simulink model "VehicleDynamics3D"  (R2019b)
settings: Solver=ode15s  StartTime=0.0  StopTime=StopTime  FixedStep=.001  MaxStep=maxStep  RelTol=relTol  AbsTol=absTol  EnableMultiTasking=on
PreLoadFcn:
  | VehicleDynamicsInitialization
model workspace: external: MATLAB File sm_suspension_templates_params.m (data not in the file)
values from neighbouring files (symbols this model uses):
  followerCameraX = 7.5    [VehicleDynamicsInitialization.m]
  followerCameraZ = 3    [VehicleDynamicsInitialization.m]
  frontCameraX = -1.75    [VehicleDynamicsInitialization.m]
  frontCameraZ = 0.35    [VehicleDynamicsInitialization.m]
  isoCameraAimX = (1/2)*wheelbase    (= 0.75)    [VehicleDynamicsInitialization.m]
  isoCameraX = -3.1    [VehicleDynamicsInitialization.m]
  isoCameraY = 3.5    [VehicleDynamicsInitialization.m]
  isoCameraZ = 1.5    [VehicleDynamicsInitialization.m]
  Load = 200    [VehicleDynamicsInitialization.m]
  maxSteeringDisplacement = 10    [VehicleDynamicsInitialization.m]
  minSteeringDisplacement = -10    [VehicleDynamicsInitialization.m]
  SetPaceSampleTime = 0.1    [VehicleDynamicsInitialization.m]
  steeringInput = 0    [VehicleDynamicsInitialization.m]
  vehicleSpeed_kph = 0    [VehicleDynamicsInitialization.m]
  wheelbase = 1.5    [VehicleDynamicsInitialization.m]
undefined symbols (not defined in the file or in its folder): dwb, Floor, sigbuilder_block, wheel, X, Y, Z
libraries: sm_lib x195, sm_suspension_templates_lib x34, nesl_utility x15, Contact_Forces_Lib x4, simulink x2, fl_ps_legacy_lib x1, aerolibanimutils x1
(part 6 of 8)

== system VehicleDynamics3D/RearSuspension/L Suspension Assembly ==
  Knuckle : Subsystem  mask(Steering knuckle){H=dwb.knuckle.height, L=dwb.knuckle.length, T=dwb.knuckle.thickness, Wpr=dwb.knuckle.wheelattachprojwidth, Hpr=dwb.knuckle.wheelattachprojheight, Wc=dwb.knuckle.wishboneconnectorwidth, Rd=dwb.knuckle.driveshaftradius, Hd=dwb.knuckle.driveshaftheight, Rr=dwb.knuckle.chamferradius, Rt=dwb.knuckle.transitionradius, Rb=dwb.knuckle.ball.radius, Rp=dwb.knuckle.pin.radius, Hp=dwb.knuckle.pin.height, Ls=dwb.knuckle.steerarm.length, Ws=dwb.knuckle.steerarm.width, Ts=dwb.knuckle.steerarm.thickness, Hsf=dwb.knuckle.steerarm.forkheight, Lsf=dwb.knuckle.steerarm.forklength, Osf=dwb.knuckle.steerarm.forkoffset, Rsp=dwb.knuckle.pinradius, Rsr=dwb.knuckle.chamferradius, Rev=on, rho=dwb.knuckle.density, clr=dwb.knuckle.color}
      mask prompts: H "Height (cm):"; L "Length (cm):"; T "Thickness (cm):"; Wpr "Width of wheel attach projection (cm):"; Hpr "Height of wheel attach projection (cm):"; Wc "Width of wishbone connectors (cm):"; Rd "Drive shaft hole radius (cm):"; Hd "Drive shaft bearing housing height (cm):"; Rr "Chamfer/fillet radius (cm):"; Rt "Transition radius to wheel attach projection (cm):"; Rb "Ball radius (cm):"; Rp "Pin radius (cm):"; Hp "Pin height (cm):"; Ls "Length of arm (cm):"; Ws "Width of arm (cm):"; Ts "Thickness of arm (cm):"; Hsf "Height of forked section (cm):"; Lsf "Length of forked section (cm):"; Osf "Offset of forked section (cm):"; Rsp "Pin radius (cm):"; Rsr "Chamfer/fillet radius (cm):"; Rev "Reverse direction:"; rho "Density (kg/m^3):"; clr "Color ([r g b]):"
      mask help: This block models a steering knuckle. The wheel hub attaches to the steering knuckle. The steering knuckle attaches to the wishbone links. The ports U and D correspond to the frames where the knuckle connects to the wishbone links. The port W corresponds to the frame where the wheel hub attaches to the knuckle. The knuckle also has a rigidly attached steering arm that attaches to the steering rack via tie rods. The port S corresponds to the frame where the steering arm attaches to the tie rod.
      mask init:
      | s_knuckle_xsec = [0 -Hd/2; 0 -Hpr/2; Wpr -Hpr/2; Wpr -H/2;
      |                 Wpr+Wc -H/2; Wpr+Wc -H/2+T; Wpr+T -H/2+T;
      |                  Wpr+T -Hd/2];
      | 
      | s_knuckle_xsec = simmechanics.demohelpers.round_corners(s_knuckle_xsec, 2:7, ...
      |                              [Rr Rt Rr*ones(1,4)], 20);
      | 
      | n_knuckle_xsec = flipud([s_knuckle_xsec(:,1) -s_knuckle_xsec(:,2)]);                         
      | 
      | Roh = sqrt((L/2)^2 + (Hd/2)^2);
      | phi = atan2(Hd,L);
      | theta = linspace(pi/2-phi,pi/2+phi,50)';
      | sh_xsec = [Roh*cos(theta) Roh*sin(theta)];
      | theta = linspace(3*pi/2-phi,3*pi/2+phi,50)';
      | sh_xsec = [sh_xsec; Roh*cos(theta) Roh*sin(theta)];
      | theta = linspace(5*pi/2-phi,pi/2-phi,100)';
      | sh_xsec = [sh_xsec; sh_xsec(1,:); Rd*cos(theta) Rd*sin(theta)];
      | 
      | % Convert Rev variable into +/- 1 instead of 0 or 1
      | sgn = (2*Rev-1);
      mask DialogControl ParameterTabVar0 Prompt: Dimensions
      mask DialogControl ParameterTabVar01 Prompt: Ball
      mask DialogControl ParameterTabVar012 Prompt: Steer Arm
      mask DialogControl ParameterTabVar0123 Prompt: Material Properties
      mask Display:
      | image(imread(fullfile(matlabroot,'toolbox','physmod','sm','smdemos','suspension_templates','images','sm_isuspension_knuckle.png')));
      | port_label('RConn',1,'U');
      | port_label('RConn',2,'D');
      | port_label('LConn',1,'W');
  Lower Wishbone : sm_suspension_templates_lib/Lower Wishbone  L1=dwb.lwb.longlength  L2=dwb.lwb.shortlength  L3=dwb.lwb.wheellinklength  W3=dwb.lwb.wheellinkwidth  W=dwb.lwb.width  T=dwb.lwb.thickness  Rb=dwb.lwb.baseradius  Ob=dwb.lwb.basearcoffset  Rev=on  Lb=dwb.lwb.bracket.length  Rsh=dwb.lwb.bracket.radius  Rs=dwb.lwb.socket.radius  Hi=dwb.lwb.socket.height  Rh=dwb.lwb.socket.holeradius  Oh=dwb.lwb.socket.holeoffset  Odb=dwb.lwb.damperbracket.offset  Wdb=dwb.lwb.damperbracket.width  Ldb=dwb.lwb.damperbracket.length  Tdb=dwb.lwb.damperbracket.thickness  Sdb=dwb.lwb.damperbracket.spacing  Rhdb=dwb.lwb.damperbracket.holeradius  rho=dwb.lwb.density  clr=dwb.lwb.color
  SW Damp Joint : sm_lib/Joints/Revolute Joint  JointMode=Normal  SenseConstraintForce=off  SenseConstraintForceX=off  SenseConstraintForceY=off  SenseConstraintForceZ=off  SenseConstraintTorque=off  SenseConstraintTorqueX=off  SenseConstraintTorqueY=off  SenseConstraintTorqueZ=off  SenseTotalForce=off  SenseTotalForceX=off  SenseTotalForceY=off  SenseTotalForceZ=off  SenseTotalTorque=off  SenseTotalTorqueX=off  SenseTotalTorqueY=off  SenseTotalTorqueZ=off  CompositeWrenchDir=FollowerOnBase  CompositeWrenchFrame=BaseFrame  EquilibriumPosition=0  EquilibriumPositionUnits=deg  SpringStiffness=0  SpringStiffnessUnits=N*m/deg  DampingCoefficient=0  DampingCoefficientUnits=N*m/(deg/s)  TorqueActuationMode=NoTorque  MotionActuationMode=ComputedMotion  SensePosition=off  SenseVelocity=off  SenseAcceleration=off  SenseTorqueForce=off  SenseLowerLimitTorqueForce=off  SenseUpperLimitTorqueForce=off  LowerLimitSpecify=off  LowerLimitBound=-90  LowerLimitBoundUnits=deg  LowerLimitStiffness=1e4  LowerLimitStiffnessUnits=N*m/deg  LowerLimitDamping=10  LowerLimitDampingUnits=N*m/(deg/s)  LowerLimitTransitionRegionWidth=0.1  LowerLimitTransitionRegionWidthUnits=deg  UpperLimitSpecify=off  UpperLimitBound=90  UpperLimitBoundUnits=deg  UpperLimitStiffness=1e4  UpperLimitStiffnessUnits=N*m/deg  UpperLimitDamping=10  UpperLimitDampingUnits=N*m/(deg/s)  UpperLimitTransitionRegionWidth=0.1  UpperLimitTransitionRegionWidthUnits=deg  PositionTargetSpecify=off  PositionTargetPriority=Low  PositionTargetValue=-30  PositionTargetValueUnits=deg  VelocityTargetSpecify=off  VelocityTargetPriority=High  VelocityTargetValue=0  VelocityTargetValueUnits=deg/s
  Subsystem : Subsystem
  Subsystem1 : Subsystem
  Upper Wishbone : sm_suspension_templates_lib/Wishbone  L1=dwb.uwb.longlength  L2=dwb.uwb.shortlength  L3=dwb.uwb.wheellinklength  W3=dwb.uwb.wheellinkwidth  W=dwb.uwb.width  T=dwb.uwb.thickness  Rb=dwb.uwb.baseradius  Ob=dwb.uwb.basearcoffset  Rev=on  Lb=dwb.uwb.bracket.length  Rsh=dwb.uwb.bracket.radius  Rs=dwb.uwb.socket.radius  Hi=dwb.uwb.socket.height  Rh=dwb.uwb.socket.ballradius  Oh=dwb.uwb.socket.offset  rho=dwb.uwb.density  clr=dwb.uwb.color
  UA : PMIOPort  Side=Right
  UB : PMIOPort  Port=2  Side=Right
  T : PMIOPort  Port=3  Side=Left
  DP : PMIOPort  Port=4  Side=Right
  DA : PMIOPort  Port=5  Side=Right
  DB : PMIOPort  Port=6  Side=Right
  connections:
  Lower Wishbone/RConn1 -- Subsystem1/RConn1
  Knuckle/LConn1 -- T/RConn1
  Lower Wishbone/LConn3 -- DB/RConn1
  Lower Wishbone/LConn2 -- DA/RConn1
  Upper Wishbone/LConn1 -- UA/RConn1
  UB/RConn1 -- Upper Wishbone/LConn2
  Knuckle/RConn2 -- Subsystem1/LConn1
  SW Damp Joint/LConn1 -- Lower Wishbone/LConn1
  SW Damp Joint/RConn1 -- DP/RConn1
  Upper Wishbone/RConn1 -- Subsystem/RConn1
  Knuckle/RConn1 -- Subsystem/LConn1

== system VehicleDynamics3D/RearSuspension/R Spr-Damp Assm ==
  Cyl Bracket : sm_suspension_templates_lib/Single Bracket  L=Lb  W=Wb  T=Tb  Rh=Rbh  rho=rho  clr=cclr
  Cyl Bracket XForm : sm_lib/Frames and Transforms/Rigid Transform  TranslationMethod=StandardAxis  TranslationStandardOffset=Lc/2  TranslationLengthUnit=cm  TranslationStandardAxis=-Z  TranslationCartesianOffset=[0 0 0]  TranslationROffset=0  TranslationROffsetUnits=m  TranslationZOffset=0  TranslationZOffsetUnits=m  TranslationThetaOffset=0  TranslationThetaOffsetUnits=deg  RotationMethod=AlignedAxes  RotationAngleUnits=deg  RotationStandardAxis=+Z  RotationAngle=0  RotationArbitraryAxis=[0 0 1]  FollAlignAxisA=+Z  BaseAlignAxisA=-Z  FollAlignAxisB=+X  BaseAlignAxisB=-X  RotationSequenceAxes=FollowerAxes  RotationSequence=XYX  RotationSequenceAngles=[0 0 0]  RotationSequenceAnglesUnits=deg  RotationMatrix=[1 0 0; 0 1 0; 0 0 1]
  Cyl-Piston Joint : sm_lib/Joints/Prismatic Joint  JointMode=Normal  SenseConstraintForce=off  SenseConstraintForceX=off  SenseConstraintForceY=off  SenseConstraintForceZ=off  SenseConstraintTorque=off  SenseConstraintTorqueX=off  SenseConstraintTorqueY=off  SenseConstraintTorqueZ=off  SenseTotalForce=off  SenseTotalForceX=off  SenseTotalForceY=off  SenseTotalForceZ=off  SenseTotalTorque=off  SenseTotalTorqueX=off  SenseTotalTorqueY=off  SenseTotalTorqueZ=off  CompositeWrenchDir=FollowerOnBase  CompositeWrenchFrame=BaseFrame  EquilibriumPosition=Ls-(Lc-Lp)/2  EquilibriumPositionUnits=cm  SpringStiffness=Ks  SpringStiffnessUnits=N/m  DampingCoefficient=Kb  DampingCoefficientUnits=N/(m/s)  TorqueActuationMode=NoTorque  MotionActuationMode=ComputedMotion  SensePosition=on  SenseVelocity=off  SenseAcceleration=off  SenseTorqueForce=off  SenseLowerLimitTorqueForce=off  SenseUpperLimitTorqueForce=off  LowerLimitSpecify=off  LowerLimitBound=-1  LowerLimitBoundUnits=m  LowerLimitStiffness=1e6  LowerLimitStiffnessUnits=N/m  LowerLimitDamping=1e3  LowerLimitDampingUnits=N/(m/s)  LowerLimitTransitionRegionWidth=1e-4  LowerLimitTransitionRegionWidthUnits=m  UpperLimitSpecify=off  UpperLimitBound=1  UpperLimitBoundUnits=m  UpperLimitStiffness=1e6  UpperLimitStiffnessUnits=N/m  UpperLimitDamping=1e3  UpperLimitDampingUnits=N/(m/s)  UpperLimitTransitionRegionWidth=1e-4  UpperLimitTransitionRegionWidthUnits=m  PositionTargetSpecify=off  PositionTargetPriority=Low  PositionTargetValue=Lp/2  PositionTargetValueUnits=cm  VelocityTargetSpecify=off  VelocityTargetPriority=High  VelocityTargetValue=0  VelocityTargetValueUnits=m/s
  Cylinder : sm_lib/Body Elements/Revolved Solid  GraphicAmbientColor=[0.15 0.15 0.15 1.0]  BasedOnType=Density  CenterOfMass=[0 0 0]  CenterOfMassUnits=m  GraphicDiffuseColor=cclr  Density=rho  DensityUnits=kg/(m^3)  DoExposeReferenceFrame=on  GraphicEmissiveColor=[0.0 0.0 0.0 1.0]  ExportEntireGeometry=off  SerializedFrames=<Frames/>  MarkerShape=Sphere  MarkerSize=10  GraphicType=FromGeometry  InertiaType=CalculateFromGeometry  Mass=1  MassUnits=kg  MomentsOfInertia=[1 1 1]  MomentsOfInertiaUnits=kg*m^2  GraphicOpacity=0.75  ProductsOfInertia=[0 0 0]  ProductsOfInertiaUnits=kg*m^2  RevolutionCrossSection=cyl_xsec  RevolutionCrossSectionUnits=cm  RevolutionAngle=180  RevolutionAngleUnits=deg  RevolutionExtent=Full  GraphicShininess=75  GraphicSpecularColor=[0.5 0.5 0.5 1.0]  GraphicVisPropType=SimpleVisualProperties
      settings: SourceProductName=Simscape Multibody
  PS-Simulink Converter : nesl_utility/PS-Simulink Converter  PhysicalDomain=network_engine_domain  SubClassName=ps_output  LeftPortType=input  RightPortType=output  PseudoPeriodic=off  Frequencies=[]  Unit=cm  AffineConversion=off
  Pistion Bracket : sm_suspension_templates_lib/Single Bracket  L=Lb  W=Wb  T=Tb  Rh=Rbh  rho=rho  clr=pclr
  Piston : sm_lib/Body Elements/Revolved Solid  GraphicAmbientColor=[0.15 0.15 0.15 1.0]  BasedOnType=Density  CenterOfMass=[0 0 0]  CenterOfMassUnits=m  GraphicDiffuseColor=pclr  Density=rho  DensityUnits=kg/(m^3)  DoExposeReferenceFrame=on  GraphicEmissiveColor=[0.0 0.0 0.0 1.0]  ExportEntireGeometry=off  SerializedFrames=<Frames/>  MarkerShape=Sphere  MarkerSize=10  GraphicType=FromGeometry  InertiaType=CalculateFromGeometry  Mass=1  MassUnits=kg  MomentsOfInertia=[1 1 1]  MomentsOfInertiaUnits=kg*m^2  GraphicOpacity=1  ProductsOfInertia=[0 0 0]  ProductsOfInertiaUnits=kg*m^2  RevolutionCrossSection=piston_xsec  RevolutionCrossSectionUnits=cm  RevolutionAngle=180  RevolutionAngleUnits=deg  RevolutionExtent=Full  GraphicShininess=75  GraphicSpecularColor=[0.5 0.5 0.5 1.0]  GraphicVisPropType=SimpleVisualProperties
      settings: SourceProductName=Simscape Multibody
  Piston Bracket XForm : sm_lib/Frames and Transforms/Rigid Transform  TranslationMethod=StandardAxis  TranslationStandardOffset=Lp/2  TranslationLengthUnit=cm  TranslationStandardAxis=+Z  TranslationCartesianOffset=[0 0 0]  TranslationROffset=0  TranslationROffsetUnits=m  TranslationZOffset=0  TranslationZOffsetUnits=m  TranslationThetaOffset=0  TranslationThetaOffsetUnits=deg  RotationMethod=None  RotationAngleUnits=deg  RotationStandardAxis=+Z  RotationAngle=0  RotationArbitraryAxis=[0 0 1]  FollAlignAxisA=+Z  BaseAlignAxisA=+Z  FollAlignAxisB=+X  BaseAlignAxisB=-X  RotationSequenceAxes=FollowerAxes  RotationSequence=XYX  RotationSequenceAngles=[0 0 0]  RotationSequenceAnglesUnits=deg  RotationMatrix=[1 0 0; 0 1 0; 0 0 1]
  Terminator : Terminator
  P : PMIOPort  Side=Right
  C : PMIOPort  Port=2  Side=Left
  wires:
  PS-Simulink Converter/1 -> Terminator/1  "RRSuspensionTravel_cm"
  connections:
  C/RConn1 -- Cyl Bracket/LConn1
  Pistion Bracket/LConn1 -- P/RConn1
  Pistion Bracket/RConn1 -- Piston Bracket XForm/RConn1
  Cyl Bracket/RConn1 -- Cyl Bracket XForm/RConn1
  Cyl-Piston Joint/RConn1 -- Piston/RConn1 -- Piston Bracket XForm/LConn1
  Cylinder/RConn1 -- Cyl-Piston Joint/LConn1 -- Cyl Bracket XForm/LConn1
  Cyl-Piston Joint/RConn2 -- PS-Simulink Converter/LConn1

== system VehicleDynamics3D/RearSuspension/R Suspension Assembly ==
  Knuckle : Subsystem  mask(Steering knuckle){H=dwb.knuckle.height, L=dwb.knuckle.length, T=dwb.knuckle.thickness, Wpr=dwb.knuckle.wheelattachprojwidth, Hpr=dwb.knuckle.wheelattachprojheight, Wc=dwb.knuckle.wishboneconnectorwidth, Rd=dwb.knuckle.driveshaftradius, Hd=dwb.knuckle.driveshaftheight, Rr=dwb.knuckle.chamferradius, Rt=dwb.knuckle.transitionradius, Rb=dwb.knuckle.ball.radius, Rp=dwb.knuckle.pin.radius, Hp=dwb.knuckle.pin.height, Ls=dwb.knuckle.steerarm.length, Ws=dwb.knuckle.steerarm.width, Ts=dwb.knuckle.steerarm.thickness, Hsf=dwb.knuckle.steerarm.forkheight, Lsf=dwb.knuckle.steerarm.forklength, Osf=dwb.knuckle.steerarm.forkoffset, Rsp=dwb.knuckle.pinradius, Rsr=dwb.knuckle.chamferradius, Rev=off, rho=dwb.knuckle.density, clr=dwb.knuckle.color}
      mask prompts: H "Height (cm):"; L "Length (cm):"; T "Thickness (cm):"; Wpr "Width of wheel attach projection (cm):"; Hpr "Height of wheel attach projection (cm):"; Wc "Width of wishbone connectors (cm):"; Rd "Drive shaft hole radius (cm):"; Hd "Drive shaft bearing housing height (cm):"; Rr "Chamfer/fillet radius (cm):"; Rt "Transition radius to wheel attach projection (cm):"; Rb "Ball radius (cm):"; Rp "Pin radius (cm):"; Hp "Pin height (cm):"; Ls "Length of arm (cm):"; Ws "Width of arm (cm):"; Ts "Thickness of arm (cm):"; Hsf "Height of forked section (cm):"; Lsf "Length of forked section (cm):"; Osf "Offset of forked section (cm):"; Rsp "Pin radius (cm):"; Rsr "Chamfer/fillet radius (cm):"; Rev "Reverse direction:"; rho "Density (kg/m^3):"; clr "Color ([r g b]):"
      mask help: This block models a steering knuckle. The wheel hub attaches to the steering knuckle. The steering knuckle attaches to the wishbone links. The ports U and D correspond to the frames where the knuckle connects to the wishbone links. The port W corresponds to the frame where the wheel hub attaches to the knuckle. The knuckle also has a rigidly attached steering arm that attaches to the steering rack via tie rods. The port S corresponds to the frame where the steering arm attaches to the tie rod.
      mask init: same as VehicleDynamics3D/RearSuspension/L Suspension Assembly/Knuckle
      mask DialogControl ParameterTabVar0 Prompt: Dimensions
      mask DialogControl ParameterTabVar01 Prompt: Ball
      mask DialogControl ParameterTabVar012 Prompt: Steer Arm
      mask DialogControl ParameterTabVar0123 Prompt: Material Properties
      mask Display:
      | image(imread(fullfile(matlabroot,'toolbox','physmod','sm','smdemos','suspension_templates','images','sm_isuspension_knuckle.png')));
      | port_label('RConn',1,'U');
      | port_label('RConn',2,'D');
      | port_label('LConn',1,'W');
  Lower Wishbone : sm_suspension_templates_lib/Lower Wishbone  L1=dwb.lwb.longlength  L2=dwb.lwb.shortlength  L3=dwb.lwb.wheellinklength  W3=dwb.lwb.wheellinkwidth  W=dwb.lwb.width  T=dwb.lwb.thickness  Rb=dwb.lwb.baseradius  Ob=dwb.lwb.basearcoffset  Rev=off  Lb=dwb.lwb.bracket.length  Rsh=dwb.lwb.bracket.radius  Rs=dwb.lwb.socket.radius  Hi=dwb.lwb.socket.height  Rh=dwb.lwb.socket.holeradius  Oh=dwb.lwb.socket.holeoffset  Odb=dwb.lwb.damperbracket.offset  Wdb=dwb.lwb.damperbracket.width  Ldb=dwb.lwb.damperbracket.length  Tdb=dwb.lwb.damperbracket.thickness  Sdb=dwb.lwb.damperbracket.spacing  Rhdb=dwb.lwb.damperbracket.holeradius  rho=dwb.lwb.density  clr=dwb.lwb.color
  SE Damp Joint : sm_lib/Joints/Revolute Joint  JointMode=Normal  SenseConstraintForce=off  SenseConstraintForceX=off  SenseConstraintForceY=off  SenseConstraintForceZ=off  SenseConstraintTorque=off  SenseConstraintTorqueX=off  SenseConstraintTorqueY=off  SenseConstraintTorqueZ=off  SenseTotalForce=off  SenseTotalForceX=off  SenseTotalForceY=off  SenseTotalForceZ=off  SenseTotalTorque=off  SenseTotalTorqueX=off  SenseTotalTorqueY=off  SenseTotalTorqueZ=off  CompositeWrenchDir=FollowerOnBase  CompositeWrenchFrame=BaseFrame  EquilibriumPosition=0  EquilibriumPositionUnits=deg  SpringStiffness=0  SpringStiffnessUnits=N*m/deg  DampingCoefficient=0  DampingCoefficientUnits=N*m/(deg/s)  TorqueActuationMode=NoTorque  MotionActuationMode=ComputedMotion  SensePosition=off  SenseVelocity=off  SenseAcceleration=off  SenseTorqueForce=off  SenseLowerLimitTorqueForce=off  SenseUpperLimitTorqueForce=off  LowerLimitSpecify=off  LowerLimitBound=-90  LowerLimitBoundUnits=deg  LowerLimitStiffness=1e4  LowerLimitStiffnessUnits=N*m/deg  LowerLimitDamping=10  LowerLimitDampingUnits=N*m/(deg/s)  LowerLimitTransitionRegionWidth=0.1  LowerLimitTransitionRegionWidthUnits=deg  UpperLimitSpecify=off  UpperLimitBound=90  UpperLimitBoundUnits=deg  UpperLimitStiffness=1e4  UpperLimitStiffnessUnits=N*m/deg  UpperLimitDamping=10  UpperLimitDampingUnits=N*m/(deg/s)  UpperLimitTransitionRegionWidth=0.1  UpperLimitTransitionRegionWidthUnits=deg  PositionTargetSpecify=off  PositionTargetPriority=Low  PositionTargetValue=150  PositionTargetValueUnits=deg  VelocityTargetSpecify=off  VelocityTargetPriority=High  VelocityTargetValue=0  VelocityTargetValueUnits=deg/s
  Subsystem : Subsystem
  Subsystem1 : Subsystem
  Upper Wishbone : sm_suspension_templates_lib/Wishbone  L1=dwb.uwb.longlength  L2=dwb.uwb.shortlength  L3=dwb.uwb.wheellinklength  W3=dwb.uwb.wheellinkwidth  W=dwb.uwb.width  T=dwb.uwb.thickness  Rb=dwb.uwb.baseradius  Ob=dwb.uwb.basearcoffset  Rev=off  Lb=dwb.uwb.bracket.length  Rsh=dwb.uwb.bracket.radius  Rs=dwb.uwb.socket.radius  Hi=dwb.uwb.socket.height  Rh=dwb.uwb.socket.ballradius  Oh=dwb.uwb.socket.offset  rho=dwb.uwb.density  clr=dwb.uwb.color
  UA : PMIOPort  Side=Left
  UB : PMIOPort  Port=2  Side=Left
  T : PMIOPort  Port=3  Side=Right
  DP : PMIOPort  Port=4  Side=Left
  DA : PMIOPort  Port=5  Side=Left
  DB : PMIOPort  Port=6  Side=Left
  connections:
  Lower Wishbone/RConn1 -- Subsystem/LConn1
  Lower Wishbone/LConn3 -- DB/RConn1
  Lower Wishbone/LConn2 -- DA/RConn1
  UA/RConn1 -- Upper Wishbone/LConn1
  Subsystem/RConn1 -- Knuckle/RConn2
  UB/RConn1 -- Upper Wishbone/LConn2
  DP/RConn1 -- SE Damp Joint/LConn1
  SE Damp Joint/RConn1 -- Lower Wishbone/LConn1
  T/RConn1 -- Knuckle/LConn1
  Subsystem1/RConn1 -- Knuckle/RConn1
  Subsystem1/LConn1 -- Upper Wishbone/RConn1

== system VehicleDynamics3D/WheelFL/FrontLeftWeelContact ==
  Bus Selector : BusSelector  OutputSignals=Normal Force,Friction Force
  Math Function : Math  Operator=square  SaturateOnIntegerOverflow=on
  Rigid Transform : sm_lib/Frames and Transforms/Rigid Transform  TranslationMethod=StandardAxis  TranslationStandardOffset=-wheel.tire.outerradius*.01  TranslationLengthUnit=m  TranslationStandardAxis=+Z  TranslationCartesianOffset=[0 0 0]  TranslationROffset=0  TranslationROffsetUnits=m  TranslationZOffset=0  TranslationZOffsetUnits=m  TranslationThetaOffset=0  TranslationThetaOffsetUnits=deg  RotationMethod=None  RotationAngleUnits=deg  RotationStandardAxis=+Z  RotationAngle=0  RotationArbitraryAxis=[0 0 1]  FollAlignAxisA=+X  BaseAlignAxisA=-X  FollAlignAxisB=+Z  BaseAlignAxisB=+Z  RotationSequenceAxes=FollowerAxes  RotationSequence=XYX  RotationSequenceAngles=[0 0 0]  RotationSequenceAnglesUnits=deg  RotationMatrix=[1 0 0; 0 1 0; 0 0 1]
  Signal Conversion : SignalConversion  OverrideOpt=off
  Signal Conversion1 : SignalConversion  OverrideOpt=off
  Sphere to Plane Force : Contact_Forces_Lib/3D/Sphere to Plane Force  sphere_rad=wheel.tire.outerradius*.01  plane_lenx=Floor.l  plane_leny=Floor.w  plane_depth=Floor.h/2  force_law=Nonlinear  k_contact=contactStiffness  b_contact=contactDamping  pen_full_damp_F=1e-4  pen_exponent=1  custom_param_1=1  custom_param_2=1  friction_law=Stick-Slip Continuous  mu_kinetic=kineticFrictionCoeff  mu_static=staticFrictionCoeff  v_thr=velocityThreshold  vis_on=off  vis_opc_en=0  vis_len_plaBz=0.005  vis_clr=[0.9 0.2 0.2]  vis_opc=0.7
  Sqrt : Sqrt  SaturateOnIntegerOverflow=on
  Sum of Elements : Sum  Inputs=+
  Terminator : Terminator
  Terminator1 : Terminator
  Conn1 : PMIOPort  Side=Right
  Conn2 : PMIOPort  Port=2  Side=Left
  wires:
  Sphere to Plane Force/1 -> Bus Selector/1  "FrontLeft"
  Math Function/1 -> Sum of Elements/1
  Sum of Elements/1 -> Sqrt/1
  Bus Selector/2 -> Math Function/1  "<Friction Force>"
  Bus Selector/1 -> Signal Conversion/1  "<Normal Force>"
  Sqrt/1 -> Signal Conversion1/1
  Signal Conversion/1 -> Terminator/1  "FrontLeftTireLoad"
  Signal Conversion1/1 -> Terminator1/1  "FrontLeftFriction"
  connections:
  Conn2/RConn1 -- Sphere to Plane Force/RConn1
  Sphere to Plane Force/LConn1 -- Rigid Transform/LConn1
  Conn1/RConn1 -- Rigid Transform/RConn1

== system VehicleDynamics3D/WheelFR/FrontRightWeelContact ==
  Bus Selector : BusSelector  OutputSignals=Normal Force,Friction Force
  Math Function : Math  Operator=square  SaturateOnIntegerOverflow=on
  Rigid Transform : sm_lib/Frames and Transforms/Rigid Transform  TranslationMethod=StandardAxis  TranslationStandardOffset=-wheel.tire.outerradius*.01  TranslationLengthUnit=m  TranslationStandardAxis=+Z  TranslationCartesianOffset=[0 0 0]  TranslationROffset=0  TranslationROffsetUnits=m  TranslationZOffset=0  TranslationZOffsetUnits=m  TranslationThetaOffset=0  TranslationThetaOffsetUnits=deg  RotationMethod=None  RotationAngleUnits=deg  RotationStandardAxis=+Z  RotationAngle=0  RotationArbitraryAxis=[0 0 1]  FollAlignAxisA=+X  BaseAlignAxisA=-X  FollAlignAxisB=+Z  BaseAlignAxisB=+Z  RotationSequenceAxes=FollowerAxes  RotationSequence=XYX  RotationSequenceAngles=[0 0 0]  RotationSequenceAnglesUnits=deg  RotationMatrix=[1 0 0; 0 1 0; 0 0 1]
  Signal Conversion : SignalConversion  OverrideOpt=off
  Signal Conversion1 : SignalConversion  OverrideOpt=off
  Sphere to Plane Force : Contact_Forces_Lib/3D/Sphere to Plane Force  sphere_rad=wheel.tire.outerradius*.01  plane_lenx=Floor.l  plane_leny=Floor.w  plane_depth=Floor.h/2  force_law=Linear  k_contact=contactStiffness  b_contact=contactDamping  pen_full_damp_F=1e-4  pen_exponent=1  custom_param_1=1  custom_param_2=1  friction_law=Stick-Slip Continuous  mu_kinetic=kineticFrictionCoeff  mu_static=staticFrictionCoeff  v_thr=velocityThreshold  vis_on=off  vis_opc_en=0  vis_len_plaBz=0.005  vis_clr=[0.9 0.2 0.2]  vis_opc=0.7
  Sqrt : Sqrt  SaturateOnIntegerOverflow=on
  Sum of Elements : Sum  Inputs=+
  Terminator : Terminator
  Terminator1 : Terminator
  Conn1 : PMIOPort  Side=Right
  Conn2 : PMIOPort  Port=2  Side=Left
  wires:
  Sphere to Plane Force/1 -> Bus Selector/1  "FrontRight"
  Signal Conversion1/1 -> Terminator1/1  "FrontRightFriction"
  Bus Selector/1 -> Signal Conversion/1  "<Normal Force>"
  Sum of Elements/1 -> Sqrt/1
  Signal Conversion/1 -> Terminator/1  "FrontRightTireLoad"
  Math Function/1 -> Sum of Elements/1
  Bus Selector/2 -> Math Function/1  "<Friction Force>"
  Sqrt/1 -> Signal Conversion1/1
  connections:
  Conn1/RConn1 -- Rigid Transform/RConn1
  Sphere to Plane Force/LConn1 -- Rigid Transform/LConn1
  Conn2/RConn1 -- Sphere to Plane Force/RConn1

== system VehicleDynamics3D/WheelRL/RearLeftWeelContact ==
  Bus Selector : BusSelector  OutputSignals=Normal Force,Friction Force
  Math Function : Math  Operator=square  SaturateOnIntegerOverflow=on
  Rigid Transform : sm_lib/Frames and Transforms/Rigid Transform  TranslationMethod=StandardAxis  TranslationStandardOffset=-wheel.tire.outerradius*.01  TranslationLengthUnit=m  TranslationStandardAxis=+Z  TranslationCartesianOffset=[0 0 0]  TranslationROffset=0  TranslationROffsetUnits=m  TranslationZOffset=0  TranslationZOffsetUnits=m  TranslationThetaOffset=0  TranslationThetaOffsetUnits=deg  RotationMethod=None  RotationAngleUnits=deg  RotationStandardAxis=+Z  RotationAngle=0  RotationArbitraryAxis=[0 0 1]  FollAlignAxisA=+X  BaseAlignAxisA=-X  FollAlignAxisB=+Z  BaseAlignAxisB=+Z  RotationSequenceAxes=FollowerAxes  RotationSequence=XYX  RotationSequenceAngles=[0 0 0]  RotationSequenceAnglesUnits=deg  RotationMatrix=[1 0 0; 0 1 0; 0 0 1]
  Signal Conversion : SignalConversion  OverrideOpt=off
  Signal Conversion1 : SignalConversion  OverrideOpt=off
  Sphere to Plane Force : Contact_Forces_Lib/3D/Sphere to Plane Force  sphere_rad=wheel.tire.outerradius*.01  plane_lenx=Floor.l  plane_leny=Floor.w  plane_depth=Floor.h/2  force_law=Linear  k_contact=contactStiffness  b_contact=contactDamping  pen_full_damp_F=1e-4  pen_exponent=1  custom_param_1=1  custom_param_2=1  friction_law=Stick-Slip Continuous  mu_kinetic=kineticFrictionCoeff  mu_static=staticFrictionCoeff  v_thr=velocityThreshold  vis_on=off  vis_opc_en=0  vis_len_plaBz=0.005  vis_clr=[0.9 0.2 0.2]  vis_opc=0.7
  Sqrt : Sqrt  SaturateOnIntegerOverflow=on
  Sum of Elements : Sum  Inputs=+
  Terminator : Terminator
  Terminator2 : Terminator
  Conn1 : PMIOPort  Side=Right
  Conn2 : PMIOPort  Port=2  Side=Left
  wires:
  Sphere to Plane Force/1 -> Bus Selector/1
  Signal Conversion1/1 -> Terminator2/1  "RearLeftFriction"
  Sum of Elements/1 -> Sqrt/1
  Bus Selector/1 -> Signal Conversion/1  "<Normal Force>"
  Bus Selector/2 -> Math Function/1  "<Friction Force>"
  Signal Conversion/1 -> Terminator/1  "RearLeftTireLoad"
  Math Function/1 -> Sum of Elements/1
  Sqrt/1 -> Signal Conversion1/1
  connections:
  Conn1/RConn1 -- Rigid Transform/RConn1
  Sphere to Plane Force/LConn1 -- Rigid Transform/LConn1
  Sphere to Plane Force/RConn1 -- Conn2/RConn1

== system VehicleDynamics3D/WheelRR/RearRightWeelContact ==
  Bus Selector : BusSelector  OutputSignals=Normal Force,Friction Force
  Math Function : Math  Operator=square  SaturateOnIntegerOverflow=on
  Rigid Transform : sm_lib/Frames and Transforms/Rigid Transform  TranslationMethod=StandardAxis  TranslationStandardOffset=-wheel.tire.outerradius*.01  TranslationLengthUnit=m  TranslationStandardAxis=+Z  TranslationCartesianOffset=[0 0 0]  TranslationROffset=0  TranslationROffsetUnits=m  TranslationZOffset=0  TranslationZOffsetUnits=m  TranslationThetaOffset=0  TranslationThetaOffsetUnits=deg  RotationMethod=None  RotationAngleUnits=deg  RotationStandardAxis=+Z  RotationAngle=0  RotationArbitraryAxis=[0 0 1]  FollAlignAxisA=+X  BaseAlignAxisA=-X  FollAlignAxisB=+Z  BaseAlignAxisB=+Z  RotationSequenceAxes=FollowerAxes  RotationSequence=XYX  RotationSequenceAngles=[0 0 0]  RotationSequenceAnglesUnits=deg  RotationMatrix=[1 0 0; 0 1 0; 0 0 1]
  Signal Conversion : SignalConversion  OverrideOpt=off
  Signal Conversion1 : SignalConversion  OverrideOpt=off
  Sphere to Plane Force : Contact_Forces_Lib/3D/Sphere to Plane Force  sphere_rad=wheel.tire.outerradius*.01  plane_lenx=Floor.l  plane_leny=Floor.w  plane_depth=Floor.h/2  force_law=Linear  k_contact=contactStiffness  b_contact=contactDamping  pen_full_damp_F=1e-4  pen_exponent=1  custom_param_1=1  custom_param_2=1  friction_law=Stick-Slip Continuous  mu_kinetic=kineticFrictionCoeff  mu_static=staticFrictionCoeff  v_thr=velocityThreshold  vis_on=off  vis_opc_en=0  vis_len_plaBz=0.005  vis_clr=[0.9 0.2 0.2]  vis_opc=0.7
  Sqrt : Sqrt  SaturateOnIntegerOverflow=on
  Sum of Elements : Sum  Inputs=+
  Terminator1 : Terminator
  Terminator2 : Terminator
  Conn1 : PMIOPort  Side=Right
  Conn2 : PMIOPort  Port=2  Side=Left
  wires:
  Sphere to Plane Force/1 -> Bus Selector/1  "RearRight"
  Bus Selector/1 -> Signal Conversion1/1  "<Normal Force>"
  Bus Selector/2 -> Signal Conversion/1  "<Friction Force>"
  Math Function/1 -> Sum of Elements/1
  Sum of Elements/1 -> Sqrt/1
  Sqrt/1 -> Terminator2/1  "RearRightFriction"
  Signal Conversion/1 -> Math Function/1
  Signal Conversion1/1 -> Terminator1/1  "RearRightTireLoad"
  connections:
  Sphere to Plane Force/LConn1 -- Rigid Transform/LConn1
  Conn1/RConn1 -- Rigid Transform/RConn1
  Conn2/RConn1 -- Sphere to Plane Force/RConn1

== system VehicleDynamics3D/FrontSuspension/6DOF Motion/WraptTo180 ==
  Yaw : Inport
  Bias : Bias  Bias=-180
  Bias1 : Bias  Bias=180
  Constant : Constant  Value=360
  Interval Test : simulink/Logic and Bit Operations/Interval Test  IntervalClosedRight=on  uplimit=180  IntervalClosedLeft=off  lowlimit=-180  OutDataTypeStr=boolean
  Math Function : Math  Operator=mod  SaturateOnIntegerOverflow=on
  Switch : Switch  Criteria=u2 ~= 0
  NormalizedYaw : Outport
  wires:
  Bias1/1 -> Math Function/1
  Switch/1 -> NormalizedYaw/1  "VehicleYawNormalized_Deg"
  Constant/1 -> Math Function/2
  Interval Test/1 -> Switch/2
  Math Function/1 -> Bias/1
  Bias/1 -> Switch/3
  Yaw/1 -> Switch/1, Interval Test/1, Bias1/1

== system VehicleDynamics3D/FrontSuspension/Chassis Assembly/Front Frame ==
  DL XForm : sm_lib/Frames and Transforms/Rigid Transform  TranslationMethod=Cartesian  TranslationStandardOffset=0  TranslationLengthUnit=cm  TranslationStandardAxis=+Z  TranslationCartesianOffset=[swc 0]  TranslationROffset=0  TranslationROffsetUnits=m  TranslationZOffset=0  TranslationZOffsetUnits=m  TranslationThetaOffset=0  TranslationThetaOffsetUnits=deg  RotationMethod=None  RotationAngleUnits=deg  RotationStandardAxis=+Z  RotationAngle=0  RotationArbitraryAxis=[0 0 1]  FollAlignAxisA=+X  BaseAlignAxisA=-X  FollAlignAxisB=+Y  BaseAlignAxisB=-Y  RotationSequenceAxes=FollowerAxes  RotationSequence=XYX  RotationSequenceAngles=[0 0 0]  RotationSequenceAnglesUnits=deg  RotationMatrix=[1 0 0; 0 1 0; 0 0 1]
  DR XForm : sm_lib/Frames and Transforms/Rigid Transform  TranslationMethod=Cartesian  TranslationStandardOffset=0  TranslationLengthUnit=cm  TranslationStandardAxis=+Z  TranslationCartesianOffset=[sec 0]  TranslationROffset=0  TranslationROffsetUnits=m  TranslationZOffset=0  TranslationZOffsetUnits=m  TranslationThetaOffset=0  TranslationThetaOffsetUnits=deg  RotationMethod=None  RotationAngleUnits=deg  RotationStandardAxis=+Z  RotationAngle=0  RotationArbitraryAxis=[0 0 1]  FollAlignAxisA=+X  BaseAlignAxisA=+Y  FollAlignAxisB=+Y  BaseAlignAxisB=+Z  RotationSequenceAxes=FollowerAxes  RotationSequence=XYX  RotationSequenceAngles=[0 0 0]  RotationSequenceAnglesUnits=deg  RotationMatrix=[1 0 0; 0 1 0; 0 0 1]
  Frame : sm_lib/Body Elements/Extruded Solid  GraphicAmbientColor=[0.15 0.15 0.15 1.0]  BasedOnType=Density  CenterOfMass=[0 0 0]  CenterOfMassUnits=m  GraphicDiffuseColor=clr  ExtrusionCrossSection=frame_xsec  ExtrusionCrossSectionUnits=cm  Density=rho  DensityUnits=kg/(m^3)  DoExposeReferenceFrame=on  GraphicEmissiveColor=[0.0 0.0 0.0 1.0]  ExportEntireGeometry=off  ExtrusionLength=T  ExtrusionLengthUnits=cm  ExtrusionType=General  SerializedFrames=<Frames/>  MarkerShape=Sphere  MarkerSize=10  GraphicType=FromGeometry  InertiaType=CalculateFromGeometry  Mass=1  MassUnits=kg  MomentsOfInertia=[1 1 1]  MomentsOfInertiaUnits=kg*m^2  PolygonNumSides=3  GraphicOpacity=1.0  PolygonOuterRadius=1  PolygonOuterRadiusUnits=m  ProductsOfInertia=[0 0 0]  ProductsOfInertiaUnits=kg*m^2  GraphicShininess=75  GraphicSpecularColor=[0.5 0.5 0.5 1.0]  GraphicVisPropType=SimpleVisualProperties
      settings: SourceProductName=Simscape Multibody
  UL XForm : sm_lib/Frames and Transforms/Rigid Transform  TranslationMethod=Cartesian  TranslationStandardOffset=0  TranslationLengthUnit=cm  TranslationStandardAxis=+Z  TranslationCartesianOffset=[nwc 0]  TranslationROffset=0  TranslationROffsetUnits=m  TranslationZOffset=0  TranslationZOffsetUnits=m  TranslationThetaOffset=0  TranslationThetaOffsetUnits=deg  RotationMethod=None  RotationAngleUnits=deg  RotationStandardAxis=+Z  RotationAngle=0  RotationArbitraryAxis=[0 0 1]  FollAlignAxisA=+X  BaseAlignAxisA=-X  FollAlignAxisB=+Y  BaseAlignAxisB=-Y  RotationSequenceAxes=FollowerAxes  RotationSequence=XYX  RotationSequenceAngles=[0 0 0]  RotationSequenceAnglesUnits=deg  RotationMatrix=[1 0 0; 0 1 0; 0 0 1]
  UR XForm : sm_lib/Frames and Transforms/Rigid Transform  TranslationMethod=Cartesian  TranslationStandardOffset=0  TranslationLengthUnit=cm  TranslationStandardAxis=+Z  TranslationCartesianOffset=[nec 0]  TranslationROffset=0  TranslationROffsetUnits=m  TranslationZOffset=0  TranslationZOffsetUnits=m  TranslationThetaOffset=0  TranslationThetaOffsetUnits=deg  RotationMethod=None  RotationAngleUnits=deg  RotationStandardAxis=+Z  RotationAngle=0  RotationArbitraryAxis=[0 0 1]  FollAlignAxisA=+X  BaseAlignAxisA=+Y  FollAlignAxisB=+Y  BaseAlignAxisB=+Z  RotationSequenceAxes=FollowerAxes  RotationSequence=XYX  RotationSequenceAngles=[0 0 0]  RotationSequenceAnglesUnits=deg  RotationMatrix=[1 0 0; 0 1 0; 0 0 1]
  UL : PMIOPort  Side=Left
  DL : PMIOPort  Port=2  Side=Left
  DR : PMIOPort  Port=3  Side=Left
  UR : PMIOPort  Port=4  Side=Left
  connections:
  Frame/RConn1 -- UL XForm/LConn1 -- DL XForm/LConn1 -- DR XForm/LConn1 -- UR XForm/LConn1
  UR XForm/RConn1 -- UR/RConn1
  DL XForm/RConn1 -- DL/RConn1
  UL XForm/RConn1 -- UL/RConn1
  DR XForm/RConn1 -- DR/RConn1

== system VehicleDynamics3D/FrontSuspension/Chassis Assembly/Load ==
  Chassis Load : sm_lib/Body Elements/Brick Solid  GraphicAmbientColor=[0.15 0.15 0.15 1.0]  BasedOnType=Mass  BrickDimensions=[5 5 5]  BrickDimensionUnits=cm  CenterOfMass=[0 0 0]  CenterOfMassUnits=m  GraphicDiffuseColor=[0.6 0.0 0.0]  Density=1000  DensityUnits=kg/(m^3)  DoExposeReferenceFrame=on  GraphicEmissiveColor=[0.0 0.0 0.0 1.0]  ExportEntireGeometry=off  SerializedFrames=<Frames/>  MarkerShape=Sphere  MarkerSize=10  GraphicType=FromGeometry  InertiaType=PointMass  Mass=Load  MassUnits=kg  MomentsOfInertia=[1 1 1]  MomentsOfInertiaUnits=kg*m^2  GraphicOpacity=1.0  ProductsOfInertia=[0 0 0]  ProductsOfInertiaUnits=kg*m^2  GraphicShininess=75  GraphicSpecularColor=[0.5 0.5 0.5 1.0]  GraphicVisPropType=SimpleVisualProperties
  Chassis Load XForm : sm_lib/Frames and Transforms/Rigid Transform  TranslationMethod=StandardAxis  TranslationStandardOffset=15  TranslationLengthUnit=cm  TranslationStandardAxis=+X  TranslationCartesianOffset=[0 0 0]  TranslationROffset=0  TranslationROffsetUnits=m  TranslationZOffset=0  TranslationZOffsetUnits=m  TranslationThetaOffset=0  TranslationThetaOffsetUnits=deg  RotationMethod=None  RotationAngleUnits=deg  RotationStandardAxis=+Z  RotationAngle=0  RotationArbitraryAxis=[0 0 1]  FollAlignAxisA=+X  BaseAlignAxisA=+Y  FollAlignAxisB=+Y  BaseAlignAxisB=+Z  RotationSequenceAxes=FollowerAxes  RotationSequence=XYX  RotationSequenceAngles=[0 0 0]  RotationSequenceAnglesUnits=deg  RotationMatrix=[1 0 0; 0 1 0; 0 0 1]
  L : PMIOPort  Side=Right
  connections:
  Chassis Load XForm/LConn1 -- L/RConn1
  Chassis Load/RConn1 -- Chassis Load XForm/RConn1

== system VehicleDynamics3D/FrontSuspension/Chassis Assembly/Steering System ==
  L Rack Bracket : sm_suspension_templates_lib/Rectangular Hole Bracket  L=dwb.chassis.steering.bracket.length  W=dwb.chassis.steering.bracket.width  T=dwb.chassis.steering.bracket.thickness  Lh=dwb.chassis.steering.bracket.holelength  Wh=dwb.chassis.steering.bracket.holewidth  Rr=dwb.chassis.steering.bracket.chamferradius  rho=dwb.chassis.steering.bracket.density  clr=dwb.chassis.steering.bracket.color
  L Rack Bracket XForm : sm_lib/Frames and Transforms/Rigid Transform  TranslationMethod=Cartesian  TranslationStandardOffset=0  TranslationLengthUnit=cm  TranslationStandardAxis=+X  TranslationCartesianOffset=[-1 -35 -18]  TranslationROffset=0  TranslationROffsetUnits=m  TranslationZOffset=0  TranslationZOffsetUnits=m  TranslationThetaOffset=0  TranslationThetaOffsetUnits=deg  RotationMethod=AlignedAxes  RotationAngleUnits=deg  RotationStandardAxis=+Z  RotationAngle=0  RotationArbitraryAxis=[0 0 1]  FollAlignAxisA=+Z  BaseAlignAxisA=-X  FollAlignAxisB=+X  BaseAlignAxisB=-Z  RotationSequenceAxes=FollowerAxes  RotationSequence=XYX  RotationSequenceAngles=[0 0 0]  RotationSequenceAnglesUnits=deg  RotationMatrix=[1 0 0; 0 1 0; 0 0 1]
  L Tie Rod : sm_suspension_templates_lib/Tie Rod  L=dwb.chassis.steering.tierod.rod.length  R=dwb.chassis.steering.tierod.rod.radius  Rr=dwb.chassis.steering.tierod.rod.chamferradius  Lb=dwb.chassis.steering.tierod.bracket.length  Wb=dwb.chassis.steering.tierod.bracket.width  Tb=dwb.chassis.steering.tierod.bracket.thickness  Sb=dwb.chassis.steering.tierod.bracket.flangespacing  Rs=dwb.chassis.steering.tierod.bracket.socketradius  Rb=dwb.chassis.steering.tierod.bracket.ballradius  Rh=dwb.chassis.steering.tierod.bracket.holeradius  rho=dwb.chassis.steering.tierod.density  tclr=dwb.chassis.steering.tierod.rod.color  bclr=dwb.chassis.steering.tierod.ballcolor
  LBR Joint : sm_lib/Joints/Prismatic Joint  JointMode=Normal  SenseConstraintForce=off  SenseConstraintForceX=off  SenseConstraintForceY=off  SenseConstraintForceZ=off  SenseConstraintTorque=off  SenseConstraintTorqueX=off  SenseConstraintTorqueY=off  SenseConstraintTorqueZ=off  SenseTotalForce=off  SenseTotalForceX=off  SenseTotalForceY=off  SenseTotalForceZ=off  SenseTotalTorque=off  SenseTotalTorqueX=off  SenseTotalTorqueY=off  SenseTotalTorqueZ=off  CompositeWrenchDir=FollowerOnBase  CompositeWrenchFrame=BaseFrame  EquilibriumPosition=0  EquilibriumPositionUnits=m  SpringStiffness=steeringJointStiffness  SpringStiffnessUnits=N/m  DampingCoefficient=steeringJointDamping  DampingCoefficientUnits=N/(m/s)  TorqueActuationMode=ComputedTorque  MotionActuationMode=InputMotion  SensePosition=off  SenseVelocity=off  SenseAcceleration=off  SenseTorqueForce=off  SenseLowerLimitTorqueForce=off  SenseUpperLimitTorqueForce=off  LowerLimitSpecify=off  LowerLimitBound=-1  LowerLimitBoundUnits=m  LowerLimitStiffness=1e6  LowerLimitStiffnessUnits=N/m  LowerLimitDamping=1e3  LowerLimitDampingUnits=N/(m/s)  LowerLimitTransitionRegionWidth=1e-4  LowerLimitTransitionRegionWidthUnits=m  UpperLimitSpecify=off  UpperLimitBound=1  UpperLimitBoundUnits=m  UpperLimitStiffness=1e6  UpperLimitStiffnessUnits=N/m  UpperLimitDamping=1e3  UpperLimitDampingUnits=N/(m/s)  UpperLimitTransitionRegionWidth=1e-4  UpperLimitTransitionRegionWidthUnits=m  PositionTargetSpecify=on  PositionTargetPriority=High  PositionTargetValue=0  PositionTargetValueUnits=cm  VelocityTargetSpecify=off  VelocityTargetPriority=High  VelocityTargetValue=0  VelocityTargetValueUnits=m/s
  LRTie Joint : sm_lib/Joints/Revolute Joint  JointMode=Normal  SenseConstraintForce=off  SenseConstraintForceX=off  SenseConstraintForceY=off  SenseConstraintForceZ=off  SenseConstraintTorque=off  SenseConstraintTorqueX=off  SenseConstraintTorqueY=off  SenseConstraintTorqueZ=off  SenseTotalForce=off  SenseTotalForceX=off  SenseTotalForceY=off  SenseTotalForceZ=off  SenseTotalTorque=off  SenseTotalTorqueX=off  SenseTotalTorqueY=off  SenseTotalTorqueZ=off  CompositeWrenchDir=FollowerOnBase  CompositeWrenchFrame=BaseFrame  EquilibriumPosition=0  EquilibriumPositionUnits=deg  SpringStiffness=0  SpringStiffnessUnits=N*m/deg  DampingCoefficient=0  DampingCoefficientUnits=N*m/(deg/s)  TorqueActuationMode=NoTorque  MotionActuationMode=ComputedMotion  SensePosition=off  SenseVelocity=off  SenseAcceleration=off  SenseTorqueForce=off  SenseLowerLimitTorqueForce=off  SenseUpperLimitTorqueForce=off  LowerLimitSpecify=off  LowerLimitBound=-90  LowerLimitBoundUnits=deg  LowerLimitStiffness=1e4  LowerLimitStiffnessUnits=N*m/deg  LowerLimitDamping=10  LowerLimitDampingUnits=N*m/(deg/s)  LowerLimitTransitionRegionWidth=0.1  LowerLimitTransitionRegionWidthUnits=deg  UpperLimitSpecify=off  UpperLimitBound=90  UpperLimitBoundUnits=deg  UpperLimitStiffness=1e4  UpperLimitStiffnessUnits=N*m/deg  UpperLimitDamping=10  UpperLimitDampingUnits=N*m/(deg/s)  UpperLimitTransitionRegionWidth=0.1  UpperLimitTransitionRegionWidthUnits=deg  PositionTargetSpecify=on  PositionTargetPriority=Low  PositionTargetValue=160  PositionTargetValueUnits=deg  VelocityTargetSpecify=off  VelocityTargetPriority=High  VelocityTargetValue=0  VelocityTargetValueUnits=deg/s
  R Rack Bracket : sm_suspension_templates_lib/Rectangular Hole Bracket  L=dwb.chassis.steering.bracket.length  W=dwb.chassis.steering.bracket.width  T=dwb.chassis.steering.bracket.thickness  Lh=dwb.chassis.steering.bracket.holelength  Wh=dwb.chassis.steering.bracket.holewidth  Rr=dwb.chassis.steering.bracket.chamferradius  rho=dwb.chassis.steering.bracket.density  clr=dwb.chassis.steering.bracket.color
  R Rack Bracket XForm : sm_lib/Frames and Transforms/Rigid Transform  TranslationMethod=Cartesian  TranslationStandardOffset=0  TranslationLengthUnit=cm  TranslationStandardAxis=-X  TranslationCartesianOffset=[-1 35 -18]  TranslationROffset=0  TranslationROffsetUnits=m  TranslationZOffset=0  TranslationZOffsetUnits=m  TranslationThetaOffset=0  TranslationThetaOffsetUnits=deg  RotationMethod=AlignedAxes  RotationAngleUnits=deg  RotationStandardAxis=+Z  RotationAngle=0  RotationArbitraryAxis=[0 0 1]  FollAlignAxisA=+Z  BaseAlignAxisA=-X  FollAlignAxisB=+X  BaseAlignAxisB=-Z  RotationSequenceAxes=FollowerAxes  RotationSequence=XYX  RotationSequenceAngles=[0 0 0]  RotationSequenceAnglesUnits=deg  RotationMatrix=[1 0 0; 0 1 0; 0 0 1]
  R Tie Rod : sm_suspension_templates_lib/Tie Rod  L=dwb.chassis.steering.tierod.rod.length  R=dwb.chassis.steering.tierod.rod.radius  Rr=dwb.chassis.steering.tierod.rod.chamferradius  Lb=dwb.chassis.steering.tierod.bracket.length  Wb=dwb.chassis.steering.tierod.bracket.width  Tb=dwb.chassis.steering.tierod.bracket.thickness  Sb=dwb.chassis.steering.tierod.bracket.flangespacing  Rs=dwb.chassis.steering.tierod.bracket.socketradius  Rb=dwb.chassis.steering.tierod.bracket.ballradius  Rh=dwb.chassis.steering.tierod.bracket.holeradius  rho=dwb.chassis.steering.tierod.density  tclr=dwb.chassis.steering.tierod.rod.color  bclr=dwb.chassis.steering.tierod.ballcolor
  RRTie Joint : sm_lib/Joints/Revolute Joint  JointMode=Normal  SenseConstraintForce=off  SenseConstraintForceX=off  SenseConstraintForceY=off  SenseConstraintForceZ=off  SenseConstraintTorque=off  SenseConstraintTorqueX=off  SenseConstraintTorqueY=off  SenseConstraintTorqueZ=off  SenseTotalForce=off  SenseTotalForceX=off  SenseTotalForceY=off  SenseTotalForceZ=off  SenseTotalTorque=off  SenseTotalTorqueX=off  SenseTotalTorqueY=off  SenseTotalTorqueZ=off  CompositeWrenchDir=FollowerOnBase  CompositeWrenchFrame=BaseFrame  EquilibriumPosition=0  EquilibriumPositionUnits=deg  SpringStiffness=0  SpringStiffnessUnits=N*m/deg  DampingCoefficient=0  DampingCoefficientUnits=N*m/(deg/s)  TorqueActuationMode=NoTorque  MotionActuationMode=ComputedMotion  SensePosition=off  SenseVelocity=off  SenseAcceleration=off  SenseTorqueForce=off  SenseLowerLimitTorqueForce=off  SenseUpperLimitTorqueForce=off  LowerLimitSpecify=off  LowerLimitBound=-90  LowerLimitBoundUnits=deg  LowerLimitStiffness=1e4  LowerLimitStiffnessUnits=N*m/deg  LowerLimitDamping=10  LowerLimitDampingUnits=N*m/(deg/s)  LowerLimitTransitionRegionWidth=0.1  LowerLimitTransitionRegionWidthUnits=deg  UpperLimitSpecify=off  UpperLimitBound=90  UpperLimitBoundUnits=deg  UpperLimitStiffness=1e4  UpperLimitStiffnessUnits=N*m/deg  UpperLimitDamping=10  UpperLimitDampingUnits=N*m/(deg/s)  UpperLimitTransitionRegionWidth=0.1  UpperLimitTransitionRegionWidthUnits=deg  PositionTargetSpecify=on  PositionTargetPriority=Low  PositionTargetValue=160  PositionTargetValueUnits=deg  VelocityTargetSpecify=off  VelocityTargetPriority=High  VelocityTargetValue=0  VelocityTargetValueUnits=deg/s
  Steer Rack : Subsystem  mask(Steering Rack){L=dwb.chassis.steering.rack.rod.length, W=dwb.chassis.steering.rack.rod.width, H=dwb.chassis.steering.rack.rod.height, Db=dwb.chassis.steering.rack.rod.bracketdistance, Rr=dwb.chassis.steering.rack.rod.chamferradius, Lb=dwb.chassis.steering.rack.bracket.length, Wb=dwb.chassis.steering.rack.bracket.width, Tb=dwb.chassis.steering.rack.bracket.thickness, Rh=dwb.chassis.steering.rack.bracket.holeradius, rho=dwb.chassis.steering.rack.density, clr=dwb.chassis.steering.rack.color}
      mask prompts: L "Length (cm):"; W "Width (cm):"; H "Height (cm):"; Db "Distance between holding brackets (cm):"; Rr "Chamfer/fillet radius (cm):"; Lb "Length (cm):"; Wb "Width (cm):"; Tb "Thickness (cm):"; Rh "Hole radius (cm):"; rho "Density (kg/m^3):"; clr "Color ([r g b]):"
      mask help: This block models a steering rack with brackets at the end that connect to tie rods. The ports LT and RT correspond to the left and right tie rod frames. The ports LB and RB refer to the left and right holding bracket frames.
      mask init:
      | rack_xsec = [W/2 -H/2; W/2 H/2; -W/2 H/2; -W/2 -H/2];
      | rack_xsec = simmechanics.demohelpers.round_corners(rack_xsec,1:4,Rr,5);
      mask DialogControl ParameterTabVar0 Prompt: Rod
      mask DialogControl ParameterTabVar01 Prompt: Brackets
      mask DialogControl ParameterTabVar012 Prompt: Material Properties
      mask Display:
      | image(imread(fullfile(matlabroot,...
      |     'toolbox','physmod','sm','smdemos',...
      |     'suspension_templates','images','sm_isuspension_steerrack.png')));
      | 
      | port_label('LConn',1,'LB');
      | port_label('LConn',2,'LT');
      | port_label('RConn',1,'RB');
      | port_label('RConn',2,'RT');
  BC : PMIOPort  Side=Left
  LT : PMIOPort  Port=2  Side=Right
  RT : PMIOPort  Port=3  Side=Right
  S : PMIOPort  Port=4  Side=Left
  connections:
  LBR Joint/RConn1 -- Steer Rack/LConn1
  R Rack Bracket/LConn1 -- R Rack Bracket XForm/RConn1
  Steer Rack/RConn2 -- RRTie Joint/LConn1
  R Tie Rod/RConn1 -- RT/RConn1
  LRTie Joint/LConn1 -- Steer Rack/LConn2
  LBR Joint/LConn1 -- L Rack Bracket/RConn1
  L Tie Rod/LConn1 -- LRTie Joint/RConn1
  LT/RConn1 -- L Tie Rod/RConn1
  RRTie Joint/RConn1 -- R Tie Rod/LConn1
  L Rack Bracket/LConn1 -- L Rack Bracket XForm/RConn1
  L Rack Bracket XForm/LConn1 -- BC/RConn1 -- R Rack Bracket XForm/LConn1
  S/RConn1 -- LBR Joint/LConn2

== system VehicleDynamics3D/Inputs/SpeedProcessing/mps2mph ==
  V[kph] : Inport
  Signal Specification : SignalSpecification  Unit=m/s
  Signal Specification1 : SignalSpecification  Unit=km/hr
  Unit Conversion : UnitConversion
  V[mps] : Outport
  wires:
  V[kph]/1 -> Signal Specification1/1
  Unit Conversion/1 -> Signal Specification/1
  Signal Specification1/1 -> Unit Conversion/1
  Signal Specification/1 -> V[mps]/1

== system VehicleDynamics3D/Inputs/User Input/Burnout ==
  note: Dummy Variables for Dashboard Instruments
  Burnout : Subsystem  Tag=STV Subsys  LoadFcn=sigbuilder_block('load');  StartFcn=sigbuilder_block('start');  StopFcn=sigbuilder_block('stop');  ClipboardFcn=sigbuilder_block('clipboard');  mask(Sigbuilder block){tuvar=[0:10]}
      mask help: Simulink:masks:SigbuilderBlock_MD
      mask init:
      | if ~strcmp(get_param(bdroot(gcbh),'SimulationStatus'),'stopped') tuvar = sigbuilder_block('maskInit'); end
      settings: CopyFcn=sigbuilder_block('copy');  DeleteFcn=sigbuilder_block('delete');  ModelCloseFcn=sigbuilder_block('modelClose');  PreSaveFcn=sigbuilder_block('preSave');  PauseFcn=sigbuilder_block('pause');  ContinueFcn=sigbuilder_block('continue');  NameChangeFcn=sigbuilder_block('namechange');  OpenFcn=sigbuilder_block('open',[-753.75 333.75 550.5 430.5 ]);  CloseFcn=sigbuilder_block('close');
      mask Display: plot(0, 0, 100, 100,[2, 2, 32, 32, 2], [68, 8, 8, 68, 68],[32, 2], [38, 38], [32, 19, 2],[53, 60, 44], [32, 17, 17, 2],[16, 16, 31, 31]);txt = getActiveGroup(gcbh);text(2, 100, txt,'verticalAlignment', 'top');
  Constant1 : Constant  Value=steeringInput
  Constant2 : Constant  Value=vehicleSpeed_kph
  Terminator : Terminator
  Terminator1 : Terminator
  Steering : Outport
  Speed : Outport  Port=2
  wires:
  Burnout/2(Speed) -> Speed/1
  Burnout/1(Steering) -> Steering/1
  Constant1/1 -> Terminator/1
  Constant2/1 -> Terminator1/1
